simulink model "MassSpringDamperSystem"  (R2019b)
settings: Solver=ode45  StartTime=0.0  StopTime=20  RelTol=1e-3
values from neighbouring files (symbols this model uses):
  b = 1    [Exercises2.m]    (also in MassSpringDamperSys.m)
  k = 1    [Exercises2.m]    (also in MassSpringDamperSys.m)
  m = 1    [Exercises2.m]    (also in MassSpringDamperSys.m)
  stepf = 10    [Exercises2.m]    (also in MassSpringDamperSys.m; RunMyModelSim.m)
  stepi = 2    [Exercises2.m]    (also in MassSpringDamperSys.m; RunMyModelSim.m = 0)
  stept = 1    [Exercises2.m]    (also in MassSpringDamperSys.m; RunMyModelSim.m)
  x0 = [0,0]    [Exercises2.m]    (also in MassSpringDamperSys.m; RunMyModelSim.m = 0)
settings Model: Creator=don  LastModifiedBy=don
settings DataIOCC: TimeSaveName=mytime

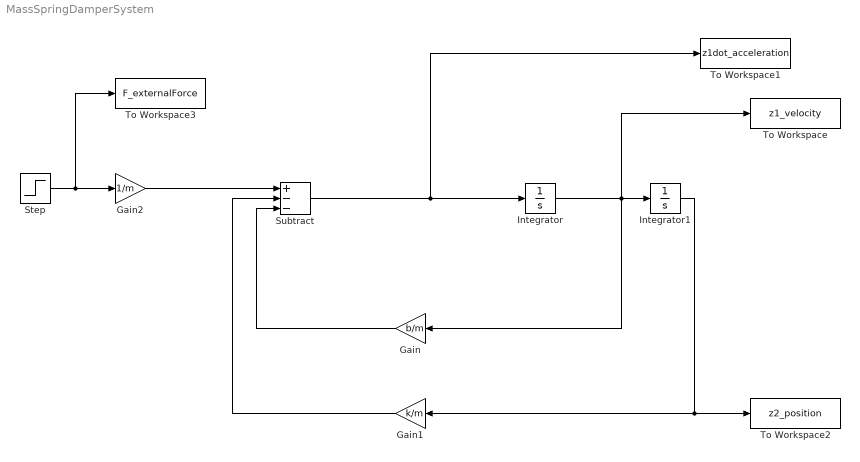
== system MassSpringDamperSystem ==
  Gain : Gain  Gain=b/m
  Gain1 : Gain  Gain=k/m
  Gain2 : Gain  Gain=1/m
  Integrator : Integrator  InitialCondition=x0
  Integrator1 : Integrator  InitialCondition=x0
  Step : Step  Time=stept  Before=stepi  After=stepf  SampleTime=0
  Subtract : Sum  Inputs=+--
  To Workspace : ToWorkspace  VariableName=z1_velocity  SampleTime=-1
  To Workspace1 : ToWorkspace  VariableName=z1dot_acceleration  SampleTime=-1
  To Workspace2 : ToWorkspace  VariableName=z2_position  SampleTime=-1
  To Workspace3 : ToWorkspace  VariableName=F_externalForce  SampleTime=-1
  wires:
  Integrator/1 -> Integrator1/1, Gain/1, To Workspace/1
  Gain/1 -> Subtract/3
  Subtract/1 -> To Workspace1/1, Integrator/1
  Integrator1/1 -> Gain1/1, To Workspace2/1
  Gain1/1 -> Subtract/2
  Step/1 -> To Workspace3/1, Gain2/1
  Gain2/1 -> Subtract/1
